simulink model "alu"  (R2024b)
settings: Solver=VariableStepAuto  StartTime=0.0  StopTime=10.0  RelTol=1e-3
libraries: simulink_extras x4
settings Model: Creator=Reon Dsouze  LastModifiedBy=Reon Dsouze

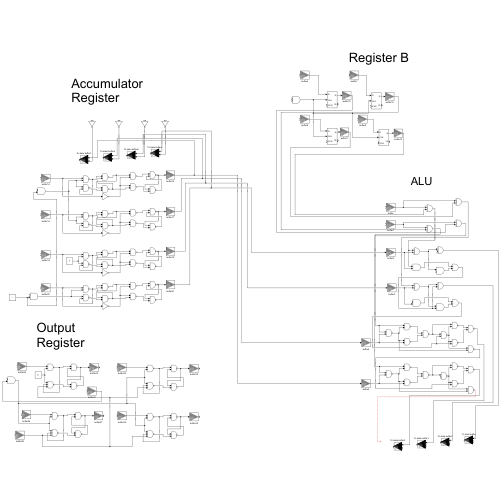
[thumbnail: Simulink's stored preview of the top-level diagram]
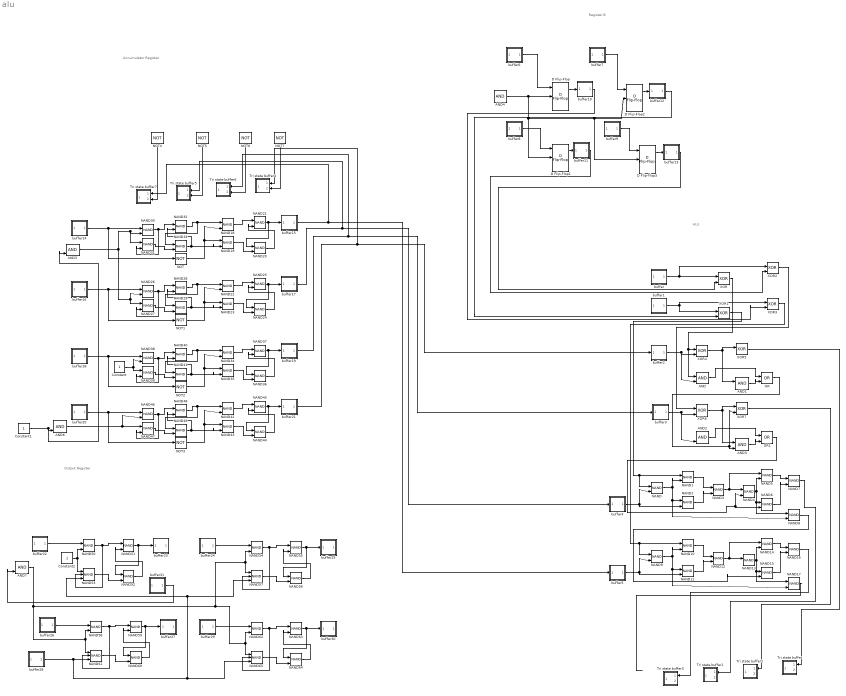
== system alu ==
  note: ALU
  note: Output Register
  note: Register B
  note: Accumulator Register
  AND{,1..7} (8 alike) : Logic  IconShape=distinctive  AllPortsSameDT=off  OutDataTypeStr=boolean
  Constant : Constant
  Constant1 : Constant
  Constant2 : Constant
  D Flip-Flop{,1..3} (4 alike) : simulink_extras/Flip Flops/D Flip-Flop
  NAND{,1..52,54..56,58..60,62..64} (62 alike) : Logic  Operator=NAND  IconShape=distinctive  AllPortsSameDT=off  OutDataTypeStr=boolean
  NAND{53,57,61,65} (4 alike) : Logic  Operator=NAND  Inputs=3  IconShape=distinctive  AllPortsSameDT=off  OutDataTypeStr=boolean
  NOT{,1..7} (8 alike) : Logic  Operator=NOT  IconShape=distinctive  AllPortsSameDT=off  OutDataTypeStr=boolean
  OR : Logic  Operator=OR  IconShape=distinctive  AllPortsSameDT=off  OutDataTypeStr=boolean
  OR1 : Logic  Operator=OR  IconShape=distinctive  AllPortsSameDT=off  OutDataTypeStr=boolean
  Tri state buffer : Subsystem
      mask Display:
      | % Draw the triangle
      | patch([1 0 1], [0 0.5 1], [0 0 0])  % Left-pointing triangle
  Tri state buffer1 : Subsystem
      mask Display:
      | % Draw the triangle
      | patch([1 0 1], [0 0.5 1], [0 0 0])  % Left-pointing triangle
  Tri state buffer2 : Subsystem
      mask Display:
      | % Draw the triangle
      | patch([1 0 1], [0 0.5 1], [0 0 0])  % Left-pointing triangle
  Tri state buffer3 : Subsystem
      mask Display:
      | % Draw the triangle
      | patch([1 0 1], [0 0.5 1], [0 0 0])  % Left-pointing triangle
  Tri state buffer4 : Subsystem
      mask Display:
      | % Draw the triangle
      | patch([1 0 1], [0 0.5 1], [0 0 0])  % Left-pointing triangle
  Tri state buffer5 : Subsystem
      mask Display:
      | % Draw the triangle
      | patch([1 0 1], [0 0.5 1], [0 0 0])  % Left-pointing triangle
  Tri state buffer6 : Subsystem
      mask Display:
      | % Draw the triangle
      | patch([1 0 1], [0 0.5 1], [0 0 0])  % Left-pointing triangle
  Tri state buffer7 : Subsystem
      mask Display:
      | % Draw the triangle
      | patch([1 0 1], [0 0.5 1], [0 0 0])  % Left-pointing triangle
  XOR{,1..7} (8 alike) : Logic  Operator=XOR  IconShape=distinctive  AllPortsSameDT=off  OutDataTypeStr=boolean
  buffer : Subsystem
      mask Display: patch([0 1 0], [0 0.5 1], [0.5 0.5 0.5]);  % This draws a triangle
  buffer1 : Subsystem
      mask Display: patch([0 1 0], [0 0.5 1], [0.5 0.5 0.5]);  % This draws a triangle
  buffer10 : Subsystem
      mask Display: patch([0 1 0], [0 0.5 1], [0.5 0.5 0.5]);  % This draws a triangle
  buffer11 : Subsystem
      mask Display: patch([0 1 0], [0 0.5 1], [0.5 0.5 0.5]);  % This draws a triangle
  buffer12 : Subsystem
      mask Display: patch([0 1 0], [0 0.5 1], [0.5 0.5 0.5]);  % This draws a triangle
  buffer13 : Subsystem
      mask Display: patch([0 1 0], [0 0.5 1], [0.5 0.5 0.5]);  % This draws a triangle
  buffer14 : Subsystem
      mask Display: patch([0 1 0], [0 0.5 1], [0.5 0.5 0.5]);  % This draws a triangle
  buffer15 : Subsystem
      mask Display: patch([0 1 0], [0 0.5 1], [0.5 0.5 0.5]);  % This draws a triangle
  buffer16 : Subsystem
      mask Display: patch([0 1 0], [0 0.5 1], [0.5 0.5 0.5]);  % This draws a triangle
  buffer17 : Subsystem
      mask Display: patch([0 1 0], [0 0.5 1], [0.5 0.5 0.5]);  % This draws a triangle
  buffer18 : Subsystem
      mask Display: patch([0 1 0], [0 0.5 1], [0.5 0.5 0.5]);  % This draws a triangle
  buffer19 : Subsystem
      mask Display: patch([0 1 0], [0 0.5 1], [0.5 0.5 0.5]);  % This draws a triangle
  buffer2 : Subsystem
      mask Display: patch([0 1 0], [0 0.5 1], [0.5 0.5 0.5]);  % This draws a triangle
  buffer20 : Subsystem
      mask Display: patch([0 1 0], [0 0.5 1], [0.5 0.5 0.5]);  % This draws a triangle
  buffer21 : Subsystem
      mask Display: patch([0 1 0], [0 0.5 1], [0.5 0.5 0.5]);  % This draws a triangle
  buffer22 : Subsystem
      mask Display: patch([0 1 0], [0 0.5 1], [0.5 0.5 0.5]);  % This draws a triangle
  buffer23 : Subsystem
      mask Display: patch([0 1 0], [0 0.5 1], [0.5 0.5 0.5]);  % This draws a triangle
  buffer24 : Subsystem
      mask Display: patch([0 1 0], [0 0.5 1], [0.5 0.5 0.5]);  % This draws a triangle
  buffer25 : Subsystem
      mask Display: patch([0 1 0], [0 0.5 1], [0.5 0.5 0.5]);  % This draws a triangle
  buffer26 : Subsystem
      mask Display: patch([0 1 0], [0 0.5 1], [0.5 0.5 0.5]);  % This draws a triangle
  buffer27 : Subsystem
      mask Display: patch([0 1 0], [0 0.5 1], [0.5 0.5 0.5]);  % This draws a triangle
  buffer28 : Subsystem
      mask Display: patch([0 1 0], [0 0.5 1], [0.5 0.5 0.5]);  % This draws a triangle
  buffer29 : Subsystem
      mask Display: patch([0 1 0], [0 0.5 1], [0.5 0.5 0.5]);  % This draws a triangle
  buffer3 : Subsystem
      mask Display: patch([0 1 0], [0 0.5 1], [0.5 0.5 0.5]);  % This draws a triangle
  buffer30 : Subsystem
      mask Display: patch([0 1 0], [0 0.5 1], [0.5 0.5 0.5]);  % This draws a triangle
  buffer31 : Subsystem
      mask Display: patch([0 1 0], [0 0.5 1], [0.5 0.5 0.5]);  % This draws a triangle
  buffer4 : Subsystem
      mask Display: patch([0 1 0], [0 0.5 1], [0.5 0.5 0.5]);  % This draws a triangle
  buffer5 : Subsystem
      mask Display: patch([0 1 0], [0 0.5 1], [0.5 0.5 0.5]);  % This draws a triangle
  buffer6 : Subsystem
      mask Display: patch([0 1 0], [0 0.5 1], [0.5 0.5 0.5]);  % This draws a triangle
  buffer7 : Subsystem
      mask Display: patch([0 1 0], [0 0.5 1], [0.5 0.5 0.5]);  % This draws a triangle
  buffer8 : Subsystem
      mask Display: patch([0 1 0], [0 0.5 1], [0.5 0.5 0.5]);  % This draws a triangle
  buffer9 : Subsystem
      mask Display: patch([0 1 0], [0 0.5 1], [0.5 0.5 0.5]);  % This draws a triangle
  wires:
  buffer/1(Out1) -> XOR2/1, XOR/1
  buffer1/1(Out1) -> XOR1/1, XOR3/1
  buffer2/1(Out1) -> AND/2, XOR4/2
  XOR4/1 -> AND1/1, XOR5/1
  AND/1 -> OR/1
  AND1/1 -> OR/2
  XOR/1 -> AND/1, XOR4/1
  AND3/1 -> OR1/2
  buffer3/1(Out1) -> AND2/2, XOR6/2
  AND2/1 -> OR1/1
  XOR6/1 -> AND3/1, XOR7/1
  OR/1 -> XOR7/2, AND3/2
  XOR2/1 -> XOR6/1
  NAND3/1 -> NAND5/1, NAND4/1
  XOR1/1 -> NAND/1, NAND1/1
  buffer4/1(Out1) -> NAND/2, NAND2/2
  NAND/1 -> NAND8/2, NAND2/1, NAND1/2
  NAND1/1 -> NAND3/1
  NAND2/1 -> NAND3/2
  NAND5/1 -> NAND7/1
  NAND4/1 -> NAND8/1, NAND6/1, NAND5/2
  NAND6/1 -> NAND7/2
  OR1/1 -> NAND4/2, NAND6/2
  NAND13/1 -> NAND17/1, NAND15/1, NAND14/2
  NAND15/1 -> NAND16/2
  buffer5/1(Out1) -> NAND9/2, NAND11/2
  NAND11/1 -> NAND12/2
  NAND9/1 -> NAND17/2, NAND11/1, NAND10/2
  NAND10/1 -> NAND12/1
  NAND14/1 -> NAND16/1
  NAND12/1 -> NAND14/1, NAND13/1
  XOR3/1 -> NAND9/1, NAND10/1
  NAND8/1 -> NAND15/2
  NAND17/1 -> ?
  NAND16/1 -> Tri state buffer3/1(In1)
  NAND7/1 -> Tri state buffer1/1(In1)
  XOR7/1 -> Tri state buffer2/1(In1)
  XOR5/1 -> Tri state buffer/1(In1)
  AND4/1 -> D Flip-Flop1/2, D Flip-Flop2/2, D Flip-Flop3/2, D Flip-Flop/2
  buffer6/1(Out1) -> D Flip-Flop/1
  buffer7/1(Out1) -> D Flip-Flop2/1
  buffer8/1(Out1) -> D Flip-Flop1/1
  buffer9/1(Out1) -> D Flip-Flop3/1
  D Flip-Flop/1 -> buffer10/1(In1)
  D Flip-Flop1/1 -> buffer11/1(In1)
  D Flip-Flop2/1 -> buffer12/1(In1)
  D Flip-Flop3/1 -> buffer13/1(In1)
  buffer10/1(Out1) -> XOR3/2
  buffer12/1(Out1) -> XOR1/2
  buffer11/1(Out1) -> XOR2/2
  buffer13/1(Out1) -> XOR/2
  NAND32/1 -> NAND33/1, NAND18/1
  NAND33/1 -> NAND32/2, NAND19/2
  buffer14/1(Out1) -> NAND30/1, NOT/1
  NOT/1 -> NAND18/2, NAND19/1
  NAND18/1 -> NAND21/1
  NAND19/1 -> NAND20/2
  NAND20/1 -> NAND21/2
  NAND21/1 -> buffer15/1(In1), NAND20/1
  NAND30/1 -> NAND31/2, NAND32/1
  NAND31/1 -> NAND33/2
  buffer16/1(Out1) -> NAND26/1, NOT1/1
  NAND25/1 -> buffer17/1(In1), NAND24/1
  NAND22/1 -> NAND25/1
  NAND26/1 -> NAND27/2, NAND28/1
  NAND27/1 -> NAND29/2
  NAND28/1 -> NAND29/1, NAND22/1
  NOT1/1 -> NAND22/2, NAND23/1
  NAND23/1 -> NAND24/2
  NAND29/1 -> NAND28/2, NAND23/2
  AND5/1 -> NAND27/1, NAND26/2, NAND31/1, NAND30/2
  NAND24/1 -> NAND25/2
  buffer18/1(Out1) -> NAND38/1, NOT2/1
  NAND37/1 -> buffer19/1(In1), NAND36/1
  NAND34/1 -> NAND37/1
  NAND41/1 -> NAND40/2, NAND35/2
  NAND35/1 -> NAND36/2
  NOT2/1 -> NAND34/2, NAND35/1
  NAND40/1 -> NAND41/1, NAND34/1
  NAND39/1 -> NAND41/2
  NAND38/1 -> NAND39/2, NAND40/1
  NAND36/1 -> NAND37/2
  NAND43/1 -> NAND44/2
  NAND49/1 -> NAND48/2, NAND43/2
  NAND47/1 -> NAND49/2
  NAND42/1 -> NAND45/1
  NAND48/1 -> NAND49/1, NAND42/1
  NAND44/1 -> NAND45/2
  NOT3/1 -> NAND42/2, NAND43/1
  NAND45/1 -> buffer21/1(In1), NAND44/1
  buffer20/1(Out1) -> NAND46/1, NOT3/1
  NAND46/1 -> NAND47/2, NAND48/1
  AND6/1 -> NAND46/2, NAND47/1
  Constant/1 -> NAND39/1, NAND38/2
  Constant1/1 -> AND5/2, AND6/2
  buffer15/1(Out1) -> buffer5/1(In1), Tri state buffer7/1(In1)
  buffer17/1(Out1) -> buffer4/1(In1), Tri state buffer5/1(In1)
  buffer19/1(Out1) -> buffer3/1(In1), Tri state buffer6/1(In1)
  buffer21/1(Out1) -> buffer2/1(In1), Tri state buffer4/1(In1)
  NOT4/1 -> Tri state buffer7/2(In2)
  NOT5/1 -> Tri state buffer5/2(In2)
  NOT6/1 -> Tri state buffer6/2(In2)
  NOT7/1 -> Tri state buffer4/2(In2)
  buffer22/1(Out1) -> NAND50/1
  Constant2/1 -> NAND50/2, NAND53/1
  NAND50/1 -> NAND53/2, NAND51/1
  NAND53/1 -> NAND52/2
  NAND51/1 -> NAND52/1, buffer23/1(In1)
  NAND52/1 -> NAND51/2
  NAND55/1 -> NAND56/1, buffer25/1(In1)
  buffer24/1(Out1) -> NAND54/1
  AND7/1 -> NAND62/2, NAND65/1, NAND57/1, NAND54/2, NAND58/2, NAND61/1
  NAND57/1 -> NAND56/2
  NAND54/1 -> NAND57/2, NAND55/1
  NAND56/1 -> NAND55/2
  NAND59/1 -> NAND60/1, buffer27/1(In1)
  buffer26/1(Out1) -> NAND58/1
  NAND61/1 -> NAND60/2
  NAND58/1 -> NAND61/2, NAND59/1
  NAND60/1 -> NAND59/2
  buffer28/1(Out1) -> NAND57/3, NAND53/3, NAND65/3, NAND61/3
  NAND64/1 -> NAND63/2
  NAND62/1 -> NAND65/2, NAND63/1
  NAND65/1 -> NAND64/2
  buffer29/1(Out1) -> NAND62/1
  NAND63/1 -> NAND64/1, buffer30/1(In1)
  buffer31/1(Out1) -> AND7/2

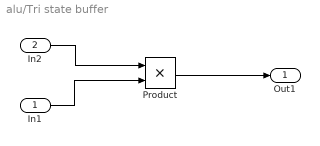
== system alu/Tri state buffer ==
  In1 : Inport
  In2 : Inport  Port=2
  Product : Product
  Out1 : Outport
  wires:
  In1/1 -> Product/2
  In2/1 -> Product/1
  Product/1 -> Out1/1

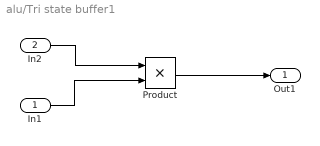
== system alu/Tri state buffer1 ==
  In1 : Inport
  In2 : Inport  Port=2
  Product : Product
  Out1 : Outport
  wires:
  In1/1 -> Product/2
  In2/1 -> Product/1
  Product/1 -> Out1/1

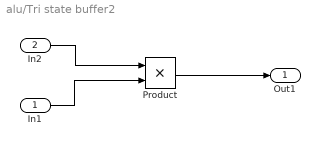
== system alu/Tri state buffer2 ==
  In1 : Inport
  In2 : Inport  Port=2
  Product : Product
  Out1 : Outport
  wires:
  In1/1 -> Product/2
  In2/1 -> Product/1
  Product/1 -> Out1/1

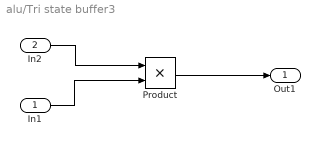
== system alu/Tri state buffer3 ==
  In1 : Inport
  In2 : Inport  Port=2
  Product : Product
  Out1 : Outport
  wires:
  In1/1 -> Product/2
  In2/1 -> Product/1
  Product/1 -> Out1/1

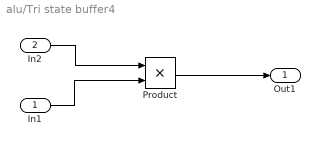
== system alu/Tri state buffer4 ==
  In1 : Inport
  In2 : Inport  Port=2
  Product : Product
  Out1 : Outport
  wires:
  In1/1 -> Product/2
  In2/1 -> Product/1
  Product/1 -> Out1/1

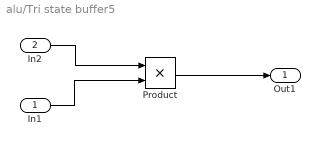
== system alu/Tri state buffer5 ==
  In1 : Inport
  In2 : Inport  Port=2
  Product : Product
  Out1 : Outport
  wires:
  In1/1 -> Product/2
  In2/1 -> Product/1
  Product/1 -> Out1/1

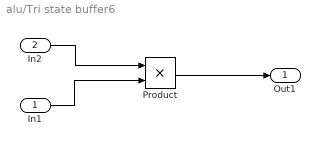
== system alu/Tri state buffer6 ==
  In1 : Inport
  In2 : Inport  Port=2
  Product : Product
  Out1 : Outport
  wires:
  In1/1 -> Product/2
  In2/1 -> Product/1
  Product/1 -> Out1/1

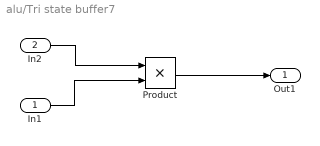
== system alu/Tri state buffer7 ==
  In1 : Inport
  In2 : Inport  Port=2
  Product : Product
  Out1 : Outport
  wires:
  In1/1 -> Product/2
  In2/1 -> Product/1
  Product/1 -> Out1/1

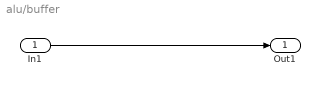
== system alu/buffer ==
  In1 : Inport
  Out1 : Outport
  wires:
  In1/1 -> Out1/1

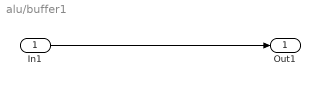
== system alu/buffer1 ==
  In1 : Inport
  Out1 : Outport
  wires:
  In1/1 -> Out1/1

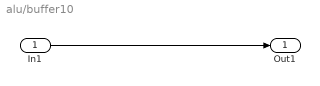
== system alu/buffer10 ==
  In1 : Inport
  Out1 : Outport
  wires:
  In1/1 -> Out1/1

== system alu/buffer11 ==
  In1 : Inport
  Out1 : Outport
  wires:
  In1/1 -> Out1/1

== system alu/buffer12 ==
  In1 : Inport
  Out1 : Outport
  wires:
  In1/1 -> Out1/1

== system alu/buffer13 ==
  In1 : Inport
  Out1 : Outport
  wires:
  In1/1 -> Out1/1

== system alu/buffer14 ==
  In1 : Inport
  Out1 : Outport
  wires:
  In1/1 -> Out1/1

== system alu/buffer15 ==
  In1 : Inport
  Out1 : Outport
  wires:
  In1/1 -> Out1/1

== system alu/buffer16 ==
  In1 : Inport
  Out1 : Outport
  wires:
  In1/1 -> Out1/1

== system alu/buffer17 ==
  In1 : Inport
  Out1 : Outport
  wires:
  In1/1 -> Out1/1

== system alu/buffer18 ==
  In1 : Inport
  Out1 : Outport
  wires:
  In1/1 -> Out1/1

== system alu/buffer19 ==
  In1 : Inport
  Out1 : Outport
  wires:
  In1/1 -> Out1/1

== system alu/buffer2 ==
  In1 : Inport
  Out1 : Outport
  wires:
  In1/1 -> Out1/1

== system alu/buffer20 ==
  In1 : Inport
  Out1 : Outport
  wires:
  In1/1 -> Out1/1

== system alu/buffer21 ==
  In1 : Inport
  Out1 : Outport
  wires:
  In1/1 -> Out1/1

== system alu/buffer22 ==
  In1 : Inport
  Out1 : Outport
  wires:
  In1/1 -> Out1/1

== system alu/buffer23 ==
  In1 : Inport
  Out1 : Outport
  wires:
  In1/1 -> Out1/1

== system alu/buffer24 ==
  In1 : Inport
  Out1 : Outport
  wires:
  In1/1 -> Out1/1

== system alu/buffer25 ==
  In1 : Inport
  Out1 : Outport
  wires:
  In1/1 -> Out1/1

== system alu/buffer26 ==
  In1 : Inport
  Out1 : Outport
  wires:
  In1/1 -> Out1/1

== system alu/buffer27 ==
  In1 : Inport
  Out1 : Outport
  wires:
  In1/1 -> Out1/1

== system alu/buffer28 ==
  In1 : Inport
  Out1 : Outport
  wires:
  In1/1 -> Out1/1

== system alu/buffer29 ==
  In1 : Inport
  Out1 : Outport
  wires:
  In1/1 -> Out1/1

== system alu/buffer3 ==
  In1 : Inport
  Out1 : Outport
  wires:
  In1/1 -> Out1/1

== system alu/buffer30 ==
  In1 : Inport
  Out1 : Outport
  wires:
  In1/1 -> Out1/1

== system alu/buffer31 ==
  In1 : Inport
  Out1 : Outport
  wires:
  In1/1 -> Out1/1

== system alu/buffer4 ==
  In1 : Inport
  Out1 : Outport
  wires:
  In1/1 -> Out1/1

== system alu/buffer5 ==
  In1 : Inport
  Out1 : Outport
  wires:
  In1/1 -> Out1/1

== system alu/buffer6 ==
  In1 : Inport
  Out1 : Outport
  wires:
  In1/1 -> Out1/1

== system alu/buffer7 ==
  In1 : Inport
  Out1 : Outport
  wires:
  In1/1 -> Out1/1

== system alu/buffer8 ==
  In1 : Inport
  Out1 : Outport
  wires:
  In1/1 -> Out1/1

== system alu/buffer9 ==
  In1 : Inport
  Out1 : Outport
  wires:
  In1/1 -> Out1/1
